simulink model "gm_ObjectTrackerHDL"  (R2024a)
settings: Solver=VariableStepAuto  StartTime=0.0  StopTime=5.5  RelTol=1e-3  EnableMultiTasking=on
PreLoadFcn:
  | % Blank input
  | img = zeros(480,640);
  | 
  | % Initialize ROI and its center
  | ROI = [175 270 127 127];
  | center = [ROI(2)+(ROI(4)+1)/2 ROI(1)+(ROI(3)+1)/2];
  | 
  | % Template Size
  | templateSize = 128;
  | tSize = templateSize;
  | 
  | % Learning rate
  | eta = 0.075;
  | 
  | % Number of training images
  | trainCount = 2;
  | 
  | % Gaussian Variance
  | sig = 2;
  | 
  | % Generate a Gaussian centered on the first frame
  | iSize = size(img);
  | [x,y] = ndgrid(1:iSize(1), 1:iSize(2));
  | gauss = exp(-((x-center(1)).^2 + (y-center(2)).^2)./(2*sig));
  | gauss = mat2gray(gauss);
  | 
  | % Generate the first template
  | img = imcrop(img, ROI);
  | gauss = imcrop(gauss, ROI);
  | 
  | % Generate the preprocess windowing function
  | [w1,w2] = meshgrid(window(@hann,tSize),window(@hann,tSize));
  | win = w1.*w2;
  | 
  | % Blank initial coefficients
  | G = zeros(tSize,tSize);
  | Ai = zeros(tSize,tSize);
  | Bi = zeros(tSize,tSize);
  | Hi = zeros(tSize,tSize);
  | 
  | numRows = tSize;
  | numCols = tSize;
InitFcn:
  | % Read the first frame
  | vidFReader = VideoReader(get_param('ObjectTrackerHDL/Input','inputFilename'));
  | img = read(vidFReader,1);
  | if (size(img,3) == 3)
  |     img = rgb2gray(img);
  | end
  | img = double(img);
  | 
  | % Initialize Object Center
  | objectCenter = str2num(get_param('ObjectTrackerHDL/ObjectTrackerHDL','objectCenter'));
  | 
  | % Template Size
  | templateSize = str2num(get_param('ObjectTrackerHDL/ObjectTrackerHDL','templateSize'));
  | originROI = objectCenter-templateSize/2;
  | tSize = templateSize;
  | 
  | % Initialize ROI and its center
  | ROI = [originROI tSize-1 tSize-1];
  | center = [ROI(2)+(ROI(4)+1)/2 ROI(1)+(ROI(3)+1)/2];
  | 
  | % Learning rate
  | eta = 0.075;
  | 
  | % Number of training images
  | trainCount = 128;
  | 
  | % Gaussian Variance
  | sig = 2;
  | 
  | % Generate a Gaussian centered on the first frame
  | iSize = size(img);
  | [x,y] = ndgrid(1:iSize(1), 1:iSize(2));
  | gauss = exp(-((x-center(1)).^2 + (y-center(2)).^2)./(2*sig));
  | gauss = mat2gray(gauss);
  | 
  | % Generate the first template
  | img = imcrop(img, ROI);
  | gauss = imcrop(gauss, ROI);
  | 
  | % Generate the preprocess windowing function
  | [w1,w2] = meshgrid(window(@hann,tSize),window(@hann,tSize));
  | win = w1.*w2;
  | 
  | % Preprocessing the first template
  | hgamma = vision.GammaCorrector(2.0,'Correction','De-gamma');
  | img = hgamma(uint8(img));
  | img = double(img);
  | mean1 = mean(img(:));
  | std1 = std(img(:));
  | img = (img-mean1)/std1;
  | fii = img.*win;
  | 
  | % Convert to frequency domain and calculate initial coefficients
  | G = fft2(gauss);
  | Ai = (G.*conj(fft2(fii)));
  | Bi = real((fft2(fii).*conj(fft2(fii))));
  | 
  | rng('default');
  | % Initial training procedure
  | for i = 1:trainCount
  |     rotateRand = 20.*rand - 10;
  |     resizeRand = 0.2.*rand + 0.9;
  |     img = imresize(imresize(imrotate(img, rotateRand), resizeRand), [tSize tSize]);
  |     img = hgamma(uint8(img));
  |     img = double(img);
  |     img = (img-mean(img(:)))/std(img(:));
  |     fii = img.*win;
  |     Ai = Ai + (G.*conj(fft2(fii)));
  |     Bi = Bi + real((fft2(fii).*conj(fft2(fii))));
  | end
  | 
  | % Initial Filter coefficients
  | Ai = eta.*Ai;
  | Bi = eta.*Bi;
  | Hi = Ai./Bi;
  | 
  | % FFT Parameters
  | numRows = tSize;
  | numCols = tSize;
model workspace (MAT data in the model file):
  mwTaskManagerKernelLatency = 0
undefined symbols (not defined in the file or in its folder): a, b, c, Rec, SDTV
libraries: hdlsllib x61, simulink x17, visionhdlutilities x8, visionstatistics x6, dsphdlxfrm2 x6, visionconversions x3, visiontransforms x3, visionhdlio x2, visionhdlconversions x2, visionhdlstatistics x2, visionsinks x1, dspvision x1
(part 1 of 3)
settings Model: SimulationMode=accelerator  Creator=The MathWorks, Inc.  LastModifiedBy=pc
settings SolverCC: PositivePriorityOrder=on
settings OptimizationCC: BlockReduction=off  ConditionallyExecuteInputs=off  DefaultParameterBehavior=Inlined  EnhancedBackFolding=on  PassReuseOutputArgsAs=Individual arguments  ZeroExternalMemoryAtStartup=off  ZeroInternalMemoryAtStartup=off  MaxStackSize=64  OptimizeBlockOrder=speed  DifferentSizesBufferReuse=on  OptimizationCustomize=off  EfficientTunableParamExpr=on
settings DebuggingCC: AlgebraicLoopMsg=error  InheritedTsInSrcMsg=none  ParameterPrecisionLossMsg=none  ParameterTunabilityLossMsg=error  FixptConstOverflowMsg=warning  SubsystemReferenceDiagnosticForUnitTest=warning
settings HardwareCC: ProdBitPerPointer=32  ProdBitPerSizeT=32  ProdBitPerPtrDiffT=32  ProdLargestAtomicFloat=None  ProdIntDivRoundTo=Undefined  ProdEndianess=Unspecified  ProdWordSize=32  ProdHWDeviceType=ASIC/FPGA->ASIC/FPGA  TargetBitPerPointer=64  TargetBitPerSizeT=64  TargetBitPerPtrDiffT=64  TargetLongLongMode=on  TargetIntDivRoundTo=Zero  TargetEndianess=LittleEndian  TargetWordSize=64  TargetHWDeviceType=Custom Processor->MATLAB Host Computer  ProdEqTarget=off  HardwareBoardFeatureSet=SoCBlockset
settings ModelReferenceCC: ModelReferenceNumInstancesAllowed=Single
settings SFSimCC: MATLABDynamicMemAlloc=off
settings RTWCC: Description=Embedded Coder  SystemTargetFile=ert.tlc  TemplateMakefile=ert_default_tmf  Toolchain=Linaro AArch64 Linux v6.3.1  GPUComputeCapability=3.5
settings CodeAppCC: ForceParamTrailComments=on  IgnoreCustomStorageClasses=off  OperatorAnnotations=on  SimulinkDataObjDesc=on  SFDataObjDesc=on  InsertBlockDesc=on
settings ERTTargetCC: ERTCustomFileTemplate=example_file_process.tlc

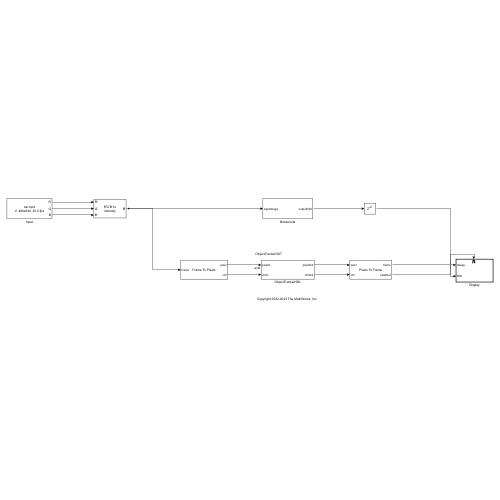
[thumbnail: Simulink's stored preview of the top-level diagram]
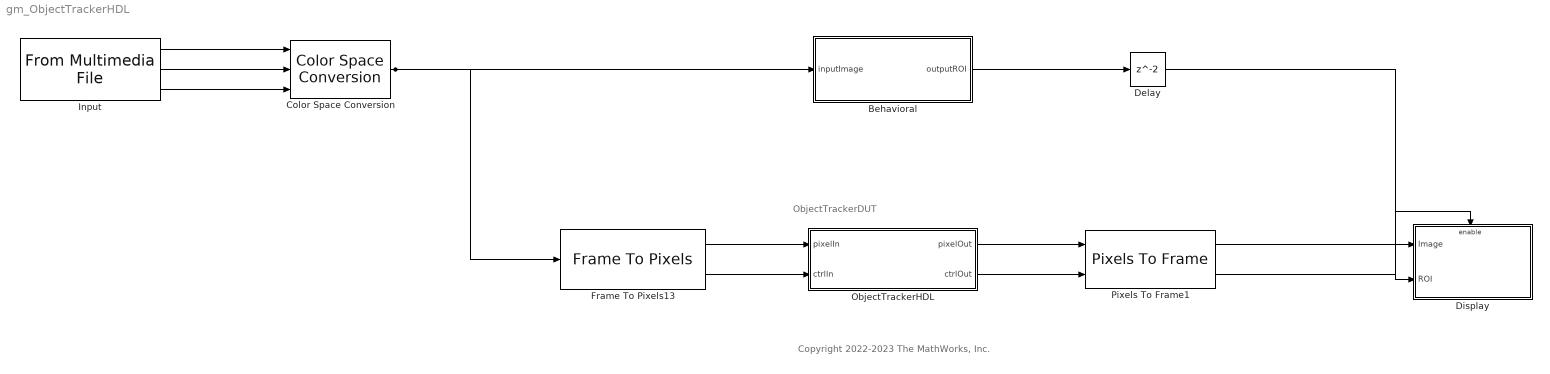
== system gm_ObjectTrackerHDL ==
  note: ObjectTrackerDUT
  note: Copyright 2022-2023 The MathWorks, Inc.
  Behavioral : Subsystem
  Color Space Conversion : visionconversions/Color Space  Conversion  conversion=Obsolete  conversionActive=R'G'B' to intensity  wp_str=D65  rec=Rec. 601 (SDTV)  sys=1125/60/2:1  imagePorts=Separate color signals
  Delay : Delay
  Display : Subsystem
  Frame To Pixels13 : visionhdlio/Frame To Pixels  NumComponents=1  NumPixels=1  VideoFormat=480p  ActivePixelsPerLine=640  ActiveVideoLines=480  TotalPixelsPerLine=800  TotalVideoLines=525  StartingActiveLine=36  FrontPorch=16  SampleTime=0  VideoFormatCache=480p  ActivePixelsPerLineCache=903  ActiveVideoLinesCache=718  TotalPixelsPerLineCache=950  TotalVideoLinesCache=750  StartingActiveLineCache=6  FrontPorchCache=5
  Input : dspvision/From Multimedia File  inputFilename=C:\Users\pc\Documents\MATLAB\Examples\R2024a\supportfiles\visionhdl\LTIR_dataset\car.mp4  readRange=[1 Inf]  loop=on  numPlays=1  outputStreams=Video only  videoDataType=uint8  audioDataType=int16  inheritSampleTime=on  userDefinedSampleTime=1  noAudioOutput=off  isIntensityVideo=off  fourcc=RGB  colorVideoFormat=Separate color signals  outputEOF=off  dataOrg=Column-major  audioFrameSize=1024  computeAudioFrameSize=off  outSamplingMode=Sample based
      settings: LibrarySourceBlock=visionsources/From Multimedia File
  ObjectTrackerHDL : Subsystem  mask{objectCenter=reshape(double([465 181]).', [1  2]), templateSize=128, imageSize=iSize}
      mask prompts: objectCenter "Object Center"; templateSize "Template Size"; imageSize "Image Size"
      mask TypeOptions templateSize: 16 | 32 | 64 | 128 | 256
  Pixels To Frame1 : visionhdlio/Pixels To Frame  NumComponents=3  NumPixels=1  VideoFormat=480p  ActivePixelsPerLine=640  ActiveVideoLines=480  TotalPixelsPerLine=800  TotalVideoLines=525  VideoFormatCache=480p  ActivePixelsPerLineCache=903  ActiveVideoLinesCache=718  TotalPixelsPerLineCache=950  TotalVideoLinesCache=750
  wires:
  Input/3 -> Color Space Conversion/3
  Input/2 -> Color Space Conversion/2
  Color Space Conversion/1 -> Frame To Pixels13/1, Behavioral/1(inputImage)
  Pixels To Frame1/1 -> Display/1(Image)
  Frame To Pixels13/2 -> ObjectTrackerHDL/2(ctrlIn)
  Input/1 -> Color Space Conversion/1
  Delay/1 -> Display/2(ROI)
  Behavioral/1(outputROI) -> Delay/1
  Pixels To Frame1/2 -> Display/Enable
  ObjectTrackerHDL/2(ctrlOut) -> Pixels To Frame1/2
  ObjectTrackerHDL/1(pixelOut) -> Pixels To Frame1/1
  Frame To Pixels13/1 -> ObjectTrackerHDL/1(pixelIn)

== system gm_ObjectTrackerHDL/Behavioral ==
  inputImage : Inport
  Preprocess : Subsystem
  Terminator : Terminator
  Track : Subsystem
  Transpose : Math  Operator=transpose
  outputROI : Outport
  wires:
  Track/2(currROI) -> Preprocess/3(currROI)
  Track/1(prevROI) -> Preprocess/2(prevROI)
  Preprocess/3(currTemplate) -> Track/2(currTemplate)
  Preprocess/2(prevTemplate) -> Track/1(prevTemplate)
  inputImage/1 -> Preprocess/1(inputImage)
  Preprocess/4(outputROI) -> Transpose/1
  Transpose/1 -> outputROI/1
  Preprocess/1(outputTemplate) -> Terminator/1

== system gm_ObjectTrackerHDL/Display ==
  Image : Inport
  ROI : Inport  Port=2
  Enable : EnablePort
  Display : visionsinks/To Video Display  windowSizeMode=True size (1:1)  openAtMdlStart=on  fullScreen=off  videoWindowX=536805376  videoWindowY=536805376  saveWindowSize=off  videoWindowWidth=1654  videoWindowHeight=1061  inputColorFormat=RGB  inputType=Obsolete  imagePorts=One multidimensional signal  OutputDevice=On-screen video monitor  dataOrg=Column-major  isWindowOpen=off
  VideoOverlay : MATLAB Function  TreatAsAtomicUnit=on
  wires:
  ROI/1 -> VideoOverlay/2(ROI)
  VideoOverlay/1(y) -> Display/1
  Image/1 -> VideoOverlay/1(img)

== system gm_ObjectTrackerHDL/ObjectTrackerHDL ==
  note: 2-D Correlation filter tracking HDL Subsystem
  pixelIn : Inport  OutDataTypeStr=uint8  PortDimensions=1  SampleTime=7.94444444444444e-08
  ctrlIn : Inport  Port=2
  Overlay : Subsystem
  Preprocess : Subsystem
  Track : Subsystem
  delayMatch : Delay  DelayLength=double(25)  InitialCondition=0  SampleTime=7.94444444444444e-08
  pixelOut : Outport  SampleTime=7.94444444444444e-08
  ctrlOut : Outport  Port=2
  wires:
  pixelIn/1 -> Overlay/1(pixelIn), Preprocess/1(pixelIn)
  ctrlIn/1 -> Overlay/2(ctrlIn), Track/5(frameCtrl), Preprocess/2(ctrlIn)
  Overlay/1(pixelOut) -> pixelOut/1
  delayMatch/1 -> ctrlOut/1
  Preprocess/5(OutputROI) -> Overlay/3(ROIIn)
  Overlay/2(ctrlOut) -> delayMatch/1
  Track/1(prevROIOut) -> Preprocess/3(prevROI)
  Track/2(currROIOut) -> Preprocess/4(currROI)
  Preprocess/1(prevPixelOut) -> Track/1(prevPixelIn)
  Preprocess/2(prevCtrlOut) -> Track/2(prevCtrlIn)
  Preprocess/3(currPixelOut) -> Track/3(currPixelIn)
  Preprocess/4(currCtrlOut) -> Track/4(currCtrlIn)

== system gm_ObjectTrackerHDL/Behavioral/Preprocess ==
  inputImage : Inport
  prevROI : Inport  Port=2
  currROI : Inport  Port=3
  Constant8 : Constant  Value=fi(win,0,16,16)  VectorParams1D=off  OutDataTypeStr=fixdt(0,16,16)  SampleTime=-1
  CurrPreprocess : Subsystem
  MATLAB Function1 : MATLAB Function  TreatAsAtomicUnit=on  mask{templateSize=tSize}
      mask prompts: templateSize "Template Size"
  MATLAB Function7 : MATLAB Function  TreatAsAtomicUnit=on  mask{templateSize=tSize}
      mask prompts: templateSize "Template Size"
  PrevPreprocess : Subsystem
  outputTemplate : Outport
  prevTemplate : Outport  Port=2
  currTemplate : Outport  Port=3
  outputROI : Outport  Port=4
  wires:
  currROI/1 -> MATLAB Function1/2(ROI)
  inputImage/1 -> MATLAB Function7/1(img), MATLAB Function1/1(img)
  prevROI/1 -> MATLAB Function7/2(ROI), outputROI/1
  PrevPreprocess/1(out) -> prevTemplate/1
  MATLAB Function1/1(fi) -> CurrPreprocess/1(in)
  Constant8/1 -> PrevPreprocess/2(window), CurrPreprocess/2(window)
  CurrPreprocess/1(out) -> currTemplate/1
  MATLAB Function7/1(fi) -> PrevPreprocess/1(in), outputTemplate/1

== system gm_ObjectTrackerHDL/Behavioral/Track ==
  prevTemplate : Inport
  currTemplate : Inport  Port=2
  2-DCorrelation : Subsystem
  MaxCorrelation : Subsystem
  ROIUpdate : Subsystem
  prevROI : Outport
  currROI : Outport  Port=2
  wires:
  2-DCorrelation/1(correlationOut) -> MaxCorrelation/1(correlationIn)
  MaxCorrelation/2(maxRow) -> ROIUpdate/2(maxRow)
  MaxCorrelation/1(maxCol) -> ROIUpdate/1(maxCol)
  prevTemplate/1 -> 2-DCorrelation/1(prevTemplate)
  ROIUpdate/1(prevROI) -> prevROI/1
  ROIUpdate/2(currROI) -> currROI/1
  currTemplate/1 -> 2-DCorrelation/2(currTemplate)

== system gm_ObjectTrackerHDL/ObjectTrackerHDL/Overlay ==
  note: Overlay Subsystem overlays the template bounding box onto the image frame
  pixelIn : Inport  OutDataTypeStr=uint8  PortDimensions=1  SampleTime=7.94444444444444e-08
  ctrlIn : Inport  Port=2
  ROIIn : Inport  Port=3  OutDataTypeStr=uint16  PortDimensions=[4]  SampleTime=7.94444444444444e-08
  Constant : Constant  OutDataTypeStr=uint16  SampleTime=7.94444444444444e-08
  ROIIn_3_term3 : Terminator
  Subtract : Sum  Inputs=+-  OutDataTypeStr=uint16  AccumDataTypeStr=uint16  SampleTime=7.94444444444444e-08
  VideoOverlay : Subsystem  mask{color=Blue, opacity=double(1), mulChannel=off, numChannel=1, planeOpacity=double(0)}
      mask prompts: opacity "Pixel Opacity"; mulChannel "Multiple Channels"; numChannel "Number of Channels"; planeOpacity "Plane Opacity"
      mask init:
      | color = double(3);
      | mulChannel = double(0);
      | numChannel = double(1);
      | opacity = double(1);
      | planeOpacity = double(0);
      mask TypeOptions color: Red | Green | Blue | Cyan | Yellow
      mask TypeOptions numChannel: 1 | 2 | 3
  concatenate : Concatenate  NumInputs=4  Mode=Multidimensional array  ConcatenateDimension=2
  t : Demux
  pixelOut : Outport  SampleTime=7.94444444444444e-08
  ctrlOut : Outport  Port=2
  wires:
  pixelIn/1 -> VideoOverlay/1(pixelIn)
  ctrlIn/1 -> VideoOverlay/2(ctrlIn)
  ROIIn/1 -> t/1
  Constant/1 -> Subtract/2
  Subtract/1 -> concatenate/4, concatenate/3
  concatenate/1 -> VideoOverlay/3(Position)
  VideoOverlay/1(pixelOut) -> pixelOut/1
  VideoOverlay/2(ctrlOut) -> ctrlOut/1
  t/1 -> concatenate/2
  t/2 -> concatenate/1
  t/3 -> Subtract/1
  t/4 -> ROIIn_3_term3/1

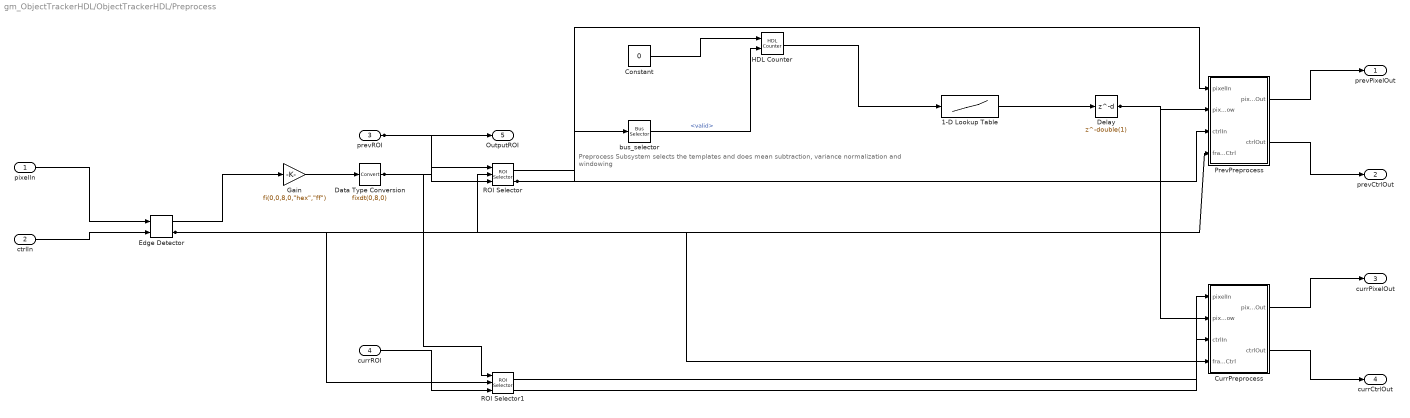
== system gm_ObjectTrackerHDL/ObjectTrackerHDL/Preprocess ==
  note: Preprocess Subsystem selects the templates and does mean subtraction, variance normalization and windowing
  pixelIn : Inport  OutDataTypeStr=uint8  PortDimensions=1  SampleTime=7.94444444444444e-08
  ctrlIn : Inport  Port=2
  prevROI : Inport  Port=3  OutDataTypeStr=uint16  PortDimensions=[4]  SampleTime=7.94444444444444e-08
  currROI : Inport  Port=4  OutDataTypeStr=uint16  PortDimensions=[4]  SampleTime=7.94444444444444e-08
  1-D Lookup Table : Lookup_n-D  NumberOfTableDimensions=1  LookupTableObject=''  BreakpointsForDimension1=[0:tSize * tSize - 1]  BreakpointsForDimension1FirstPoint=10  BreakpointsForDimension2FirstPoint=10  BreakpointsForDimension1Spacing=12  BreakpointsForDimension2Spacing=12  IndexSearchMethod=Evenly spaced points  Table=fi(win(:)',0,16,16)  InterpMethod=Flat  InternalRulePriority=Speed  OutDataTypeStr=fixdt(0,16,16)  RndMeth=Simplest
  Constant : Constant  Value=0  OutDataTypeStr=boolean  SampleTime=7.94444444444444e-08
  CurrPreprocess : Subsystem
  Data Type Conversion : DataTypeConversion  OutDataTypeStr=fixdt(0,8,0)
  Delay : Delay  DelayLength=double(1)  InitialCondition=0  SampleTime=7.94444444444444e-08
  Edge Detector : visionhdlanalysis/Edge Detector  Method=Sobel  BinaryImageOutputPort=on  GradientComponentOutputPorts=off  ThresholdSource=Property  Threshold=25  LineBufferSize=2048  PaddingMethod=Symmetric  SimulateUsing=Code generation  roundingMode=Floor  overflowMode=off  GradientMin=[]  GradientMax=[]
  Gain : Gain  Gain="fi(0,0,8,0,\"hex\",\"ff\")"  ParamDataTypeStr=fixdt(0, 8, 0)  OutDataTypeStr=uint8  SampleTime=7.94444444444444e-08
  HDL Counter : hdlsllib/Sources/HDL Counter  CountType=Count limited  CountInit=0  CountStep=1  CountMax=tSize * tSize - 1  CountFromType=Initial value  CountFrom=0  CountResetPort=on  CountLoadPort=off  CountEnbPort=on  CountDirPort=off  CountHitOutputPort=off  CountDataType=Unsigned  CountWordLen=ceil(log2(tSize * tSize - 1))  CountFracLen=0  CountSampTime=1
  PrevPreprocess : Subsystem
  ROI Selector : visionhdlutilities/ROI Selector  VerticalReuse=off  RegionsSource=Input port  NumberOfRegions=1  Regions=[100 100 50 50]  SimulateUsing=Code generation
  ROI Selector1 : visionhdlutilities/ROI Selector  VerticalReuse=off  RegionsSource=Input port  NumberOfRegions=1  Regions=[100 100 50 50]  SimulateUsing=Code generation
  bus_selector : BusSelector  OutputSignals=valid
  prevPixelOut : Outport  SampleTime=7.94444444444444e-08
  prevCtrlOut : Outport  Port=2
  currPixelOut : Outport  Port=3  SampleTime=7.94444444444444e-08
  currCtrlOut : Outport  Port=4
  OutputROI : Outport  Port=5  SampleTime=7.94444444444444e-08
  wires:
  pixelIn/1 -> Edge Detector/1
  ctrlIn/1 -> Edge Detector/2
  prevROI/1 -> OutputROI/1, ROI Selector/3
  currROI/1 -> ROI Selector1/3
  1-D Lookup Table/1 -> Delay/1
  Constant/1 -> HDL Counter/1
  CurrPreprocess/1(pixelOut) -> currPixelOut/1
  CurrPreprocess/2(ctrlOut) -> currCtrlOut/1
  Data Type Conversion/1 -> ROI Selector1/1, ROI Selector/1
  Delay/1 -> PrevPreprocess/2(pixelWindow), CurrPreprocess/2(pixelWindow)
  Edge Detector/1 -> Gain/1
  Edge Detector/2 -> PrevPreprocess/4(frameCtrl), CurrPreprocess/4(frameCtrl), ROI Selector1/2, ROI Selector/2
  Gain/1 -> Data Type Conversion/1
  HDL Counter/1 -> 1-D Lookup Table/1
  bus_selector/1 -> HDL Counter/2  "<valid>"
  PrevPreprocess/1(pixelOut) -> prevPixelOut/1
  PrevPreprocess/2(ctrlOut) -> prevCtrlOut/1
  ROI Selector/1 -> PrevPreprocess/1(pixelIn)
  ROI Selector/2 -> bus_selector/1, PrevPreprocess/3(ctrlIn)
  ROI Selector1/1 -> CurrPreprocess/1(pixelIn)
  ROI Selector1/2 -> CurrPreprocess/3(ctrlIn)

== system gm_ObjectTrackerHDL/ObjectTrackerHDL/Track ==
  note: Tracking HDL Subsystem performs 2D correlation, calculates maximum of 2D correlation point and updates the ROI
  prevPixelIn : Inport  OutDataTypeStr=fixdt(1, 32, 28)  PortDimensions=1  SampleTime=7.94444444444444e-08
  prevCtrlIn : Inport  Port=2
  currPixelIn : Inport  Port=3  OutDataTypeStr=fixdt(1, 32, 28)  PortDimensions=1  SampleTime=7.94444444444444e-08
  currCtrlIn : Inport  Port=4
  frameCtrl : Inport  Port=5
  2-DCorrelation : Subsystem
  Delay7 : Delay  DelayLength=20
  MaxCorrelation : Subsystem
  ROIUpdate : Subsystem
  prevROIOut : Outport  SampleTime=7.94444444444444e-08
  currROIOut : Outport  Port=2  SampleTime=7.94444444444444e-08
  wires:
  frameCtrl/1 -> Delay7/1, 2-DCorrelation/6(frameCtrl), MaxCorrelation/3(frameCtrl)
  ROIUpdate/2(prevROI) -> prevROIOut/1
  ROIUpdate/3(currROI) -> currROIOut/1
  2-DCorrelation/1(pixelOut) -> MaxCorrelation/1(pixelIn)
  MaxCorrelation/1(maxCol) -> ROIUpdate/1(maxCol)
  2-DCorrelation/2(ctrlOut) -> MaxCorrelation/2(ctrlIn)
  prevPixelIn/1 -> 2-DCorrelation/1(prevPixelIn)
  prevCtrlIn/1 -> 2-DCorrelation/2(prevCtrlIn)
  currPixelIn/1 -> 2-DCorrelation/3(currPixelIn)
  currCtrlIn/1 -> 2-DCorrelation/4(currCtrlIn)
  MaxCorrelation/2(maxRow) -> ROIUpdate/2(maxRow)
  ROIUpdate/1(streamCtrlOut) -> 2-DCorrelation/5(streamCtrlIn)
  Delay7/1 -> ROIUpdate/3(frameCtrl)

== system gm_ObjectTrackerHDL/Behavioral/Preprocess/CurrPreprocess ==
  in : Inport
  window : Inport  Port=2
  2-D Mean2 : visionstatistics/2-D Mean  run=off  reset_popup=None  directionMode=Entire input  dimension=1  treatSBRowAsCol=on  outputMode=Binary point scaling  outputWordLength=8  outputFracLength=0  outputLastDataTypeStr=fixdt([],8,0)  accumMode=Binary point scaling  accumWordLength=32  accumFracLength=0  accumLastDataTypeStr=fixdt([],32,0)  roiEnable=off  roiType=Rectangles  roiPortion=Entire ROI  roiOutput=Individual statistics for each ROI  roiFlag=off  roundingMode=Floor  overflowMode=on  accumDataTypeStr=fixdt([],32,0)  outputDataTypeStr=fixdt([],8,0)  outputMin=[]  outputMax=[]
  2-D Standard Deviation : visionstatistics/2-D Standard Deviation  run=off  reset_popup=None  InputProcessing=Columns as channels (frame based)  directionMode=Entire input  dimension=1  treatSBRowAsCol=on  roiEnable=off  roiType=Rectangles  roiPortion=Entire ROI  roiOutput=Individual statistics for each ROI  roiFlag=off
  Data Type Conversion2 : DataTypeConversion  OutDataTypeStr=uint8  SaturateOnIntegerOverflow=off  RndMeth=Floor
  Data Type Conversion3 : DataTypeConversion  OutDataTypeStr=single  SaturateOnIntegerOverflow=off  RndMeth=Floor
  Delay : Delay  DelayLength=1  InitialCondition=uint8(mean1)
  Delay1 : Delay  DelayLength=1  InitialCondition=uint8(std1)
  Divide1 : Product  Inputs=*/  OutDataTypeStr=fixdt(1,16,12)  SaturateOnIntegerOverflow=on
  Gamma Correction : visionconversions/Gamma Correction  operation=De-gamma  gamma=2  linearSegment=on  breakPoint=0.018
  Product : Product
  Subtract2 : Sum  Inputs=+-  OutDataTypeStr=fixdt(1,16,0)
  out : Outport
  wires:
  Delay/1 -> Subtract2/2
  Delay1/1 -> Divide1/2
  Product/1 -> out/1
  window/1 -> Product/2
  Subtract2/1 -> Divide1/1
  Data Type Conversion3/1 -> 2-D Standard Deviation/1
  2-D Mean2/1 -> Delay/1
  Divide1/1 -> Product/1
  in/1 -> Gamma Correction/1
  Data Type Conversion2/1 -> Delay1/1
  2-D Standard Deviation/1 -> Data Type Conversion2/1
  Gamma Correction/1 -> Subtract2/1, 2-D Mean2/1, Data Type Conversion3/1

== system gm_ObjectTrackerHDL/Behavioral/Preprocess/PrevPreprocess ==
  in : Inport
  window : Inport  Port=2
  2-D Mean2 : visionstatistics/2-D Mean  run=off  reset_popup=None  directionMode=Entire input  dimension=1  treatSBRowAsCol=on  outputMode=Binary point scaling  outputWordLength=8  outputFracLength=0  outputLastDataTypeStr=fixdt([],8,0)  accumMode=Binary point scaling  accumWordLength=32  accumFracLength=0  accumLastDataTypeStr=fixdt([],32,0)  roiEnable=off  roiType=Rectangles  roiPortion=Entire ROI  roiOutput=Individual statistics for each ROI  roiFlag=off  roundingMode=Floor  overflowMode=on  accumDataTypeStr=fixdt([],32,0)  outputDataTypeStr=fixdt([],8,0)  outputMin=[]  outputMax=[]
  2-D Standard Deviation : visionstatistics/2-D Standard Deviation  run=off  reset_popup=None  InputProcessing=Columns as channels (frame based)  directionMode=Entire input  dimension=1  treatSBRowAsCol=on  roiEnable=off  roiType=Rectangles  roiPortion=Entire ROI  roiOutput=Individual statistics for each ROI  roiFlag=off
  Data Type Conversion2 : DataTypeConversion  OutDataTypeStr=uint8  SaturateOnIntegerOverflow=off  RndMeth=Floor
  Data Type Conversion3 : DataTypeConversion  OutDataTypeStr=single  SaturateOnIntegerOverflow=off  RndMeth=Floor
  Delay : Delay  DelayLength=1  InitialCondition=uint8(mean1)
  Delay1 : Delay  DelayLength=1  InitialCondition=uint8(std1)
  Divide1 : Product  Inputs=*/  OutDataTypeStr=fixdt(1,16,12)  SaturateOnIntegerOverflow=on
  Gamma Correction : visionconversions/Gamma Correction  operation=De-gamma  gamma=2  linearSegment=on  breakPoint=0.018
  Product : Product
  Subtract2 : Sum  Inputs=+-  OutDataTypeStr=fixdt(1,16,0)
  out : Outport
  wires:
  Delay1/1 -> Divide1/2
  Delay/1 -> Subtract2/2
  Product/1 -> out/1
  window/1 -> Product/2
  Subtract2/1 -> Divide1/1
  Data Type Conversion3/1 -> 2-D Standard Deviation/1
  2-D Mean2/1 -> Delay/1
  Divide1/1 -> Product/1
  in/1 -> Gamma Correction/1
  Data Type Conversion2/1 -> Delay1/1
  2-D Standard Deviation/1 -> Data Type Conversion2/1
  Gamma Correction/1 -> Subtract2/1, 2-D Mean2/1, Data Type Conversion3/1

== system gm_ObjectTrackerHDL/Behavioral/Track/2-DCorrelation ==
  prevTemplate : Inport
  currTemplate : Inport  Port=2
  2-D FFT : visiontransforms/2-D FFT  TableOpt=NEW  TableOptActive=Speed  FFTImplementation=Auto  BitRevOrder=off  SkipNorm=off  firstCoeffLastDataTypeStr=Inherit: Same word length as input  outputMode=Binary point scaling  outputWordLength=24  outputFracLength=12  outputLastDataTypeStr=fixdt(1,24,12)  roundingMode=Floor  overflowMode=off  firstCoeffDataTypeStr=Inherit: Same word length as input  outputDataTypeStr=fixdt(1,24,12)  outputMin=[]  outputMax=[]
  2-D FFT1 : visiontransforms/2-D FFT  TableOpt=NEW  TableOptActive=Speed  FFTImplementation=Auto  BitRevOrder=off  SkipNorm=off  firstCoeffLastDataTypeStr=Inherit: Same word length as input  outputMode=Binary point scaling  outputWordLength=24  outputFracLength=12  outputLastDataTypeStr=fixdt(1,24,12)  roundingMode=Floor  overflowMode=off  firstCoeffDataTypeStr=Inherit: Same word length as input  outputDataTypeStr=fixdt(1,24,12)  outputMin=[]  outputMax=[]
  2-D IFFT : visiontransforms/2-D IFFT  TableOpt=NEW  TableOptActive=Speed  FFTImplementation=Auto  BitRevOrder=off  cs_in=off  divideOutput=on  SkipNorm=on  firstCoeffLastDataTypeStr=Inherit: Same word length as input  outputMode=Binary point scaling  outputWordLength=24  outputFracLength=16  outputLastDataTypeStr=fixdt(1,24,16)  roundingMode=Floor  overflowMode=off  firstCoeffDataTypeStr=Inherit: Same word length as input  outputDataTypeStr=fixdt(1,24,16)  outputMin=[]  outputMax=[]
  CoefficientsUpdate : Subsystem
  Product8 : Product  OutDataTypeStr=fixdt(1,24,16)
  Transpose : Math  Operator=transpose
  Transpose1 : Math  Operator=transpose
  Transpose2 : Math  Operator=transpose
  correlationOut : Outport
  wires:
  Transpose2/1 -> correlationOut/1
  Transpose1/1 -> CoefficientsUpdate/1(In)
  2-D FFT1/1 -> Transpose1/1
  currTemplate/1 -> 2-D FFT1/1
  Transpose/1 -> Product8/1
  2-D IFFT/1 -> Transpose2/1
  Product8/1 -> 2-D IFFT/1
  2-D FFT/1 -> Transpose/1
  CoefficientsUpdate/1(Out) -> Product8/2
  prevTemplate/1 -> 2-D FFT/1

== system gm_ObjectTrackerHDL/Behavioral/Track/MaxCorrelation ==
  correlationIn : Inport
  2-D Mean3 : visionstatistics/2-D Mean  run=off  reset_popup=None  directionMode=Entire input  dimension=1  treatSBRowAsCol=on  outputLastDataTypeStr=Inherit: Same as accumulator  accumMode=Binary point scaling  accumWordLength=16  accumFracLength=0  accumLastDataTypeStr=fixdt([],16,0)  roiEnable=off  roiType=Rectangles  roiPortion=Entire ROI  roiOutput=Individual statistics for each ROI  roiFlag=off  roundingMode=Floor  overflowMode=off  accumDataTypeStr=fixdt([],16,0)  outputDataTypeStr=Inherit: Same as accumulator  outputMin=[]  outputMax=[]
  2-D Mean4 : visionstatistics/2-D Mean  run=off  reset_popup=None  directionMode=Entire input  dimension=1  treatSBRowAsCol=on  outputLastDataTypeStr=Inherit: Same as accumulator  accumMode=Binary point scaling  accumWordLength=16  accumFracLength=0  accumLastDataTypeStr=fixdt([],16,0)  roiEnable=off  roiType=Rectangles  roiPortion=Entire ROI  roiOutput=Individual statistics for each ROI  roiFlag=off  roundingMode=Floor  overflowMode=off  accumDataTypeStr=fixdt([],16,0)  outputDataTypeStr=Inherit: Same as accumulator  outputMin=[]  outputMax=[]
  Complex to Real-Imag : ComplexToRealImag
  Data Type Conversion1 : DataTypeConversion  OutDataTypeStr=uint16  SaturateOnIntegerOverflow=off  RndMeth=Floor
  Data Type Conversion3 : DataTypeConversion  OutDataTypeStr=single  SaturateOnIntegerOverflow=off  RndMeth=Floor
  Data Type Conversion4 : DataTypeConversion  OutDataTypeStr=uint16  SaturateOnIntegerOverflow=off  RndMeth=Floor
  MATLAB Function13 : MATLAB Function  TreatAsAtomicUnit=on
  Terminator : Terminator
  maxCol : Outport
  maxRow : Outport  Port=2
  wires:
  correlationIn/1 -> Data Type Conversion3/1
  2-D Mean4/1 -> maxRow/1
  MATLAB Function13/1(P) -> Data Type Conversion1/1
  2-D Mean3/1 -> maxCol/1
  Data Type Conversion3/1 -> Complex to Real-Imag/1
  Data Type Conversion1/1 -> 2-D Mean3/1
  Data Type Conversion4/1 -> 2-D Mean4/1
  MATLAB Function13/2(Q) -> Data Type Conversion4/1
  Complex to Real-Imag/2 -> Terminator/1
  Complex to Real-Imag/1 -> MATLAB Function13/1(gi)

== system gm_ObjectTrackerHDL/Behavioral/Track/ROIUpdate ==
  maxCol : Inport
  maxRow : Inport  Port=2
  Add4 : Sum  OutDataTypeStr=uint16
  Add5 : Sum  OutDataTypeStr=uint16
  CurrValidROI : Subsystem
  Delay7 : Delay  DelayLength=1  InitialConditionSource=Input port  InitialCondition=0
      settings: InputPortMap=u0,p4
  Demux1 : Demux
  Mux1 : Mux
  PrevValidROI : Subsystem
  ROI : Constant  Value=uint16(ROI)  OutDataTypeStr=uint16  SampleTime=-1
  Subtract3 : Sum  Inputs=+-  OutDataTypeStr=fixdt(1,17,0)
  Subtract4 : Sum  Inputs=+-  OutDataTypeStr=fixdt(1,17,0)
  height/2 : Constant  Value=uint16(tSize/2)  SampleTime=-1
  width/2 : Constant  Value=uint16(tSize/2)  SampleTime=-1
  prevROI : Outport
  currROI : Outport  Port=2
  wires:
  Mux1/1 -> CurrValidROI/1(ROIIn), Delay7/1
  Delay7/1 -> Demux1/1, PrevValidROI/1(ROIIn)
  ROI/1 -> Delay7/2
  CurrValidROI/1(ROIOut) -> currROI/1
  PrevValidROI/1(ROIOut) -> prevROI/1
  maxRow/1 -> Subtract4/1
  Demux1/1 -> Add5/2
  Subtract3/1 -> Add4/1
  Add5/1 -> Mux1/1
  Add4/1 -> Mux1/2
  width/2/1 -> Subtract4/2
  Subtract4/1 -> Add5/1
  Demux1/4 -> Mux1/4
  Demux1/3 -> Mux1/3
  Demux1/2 -> Add4/2
  height/2/1 -> Subtract3/2
  maxCol/1 -> Subtract3/1

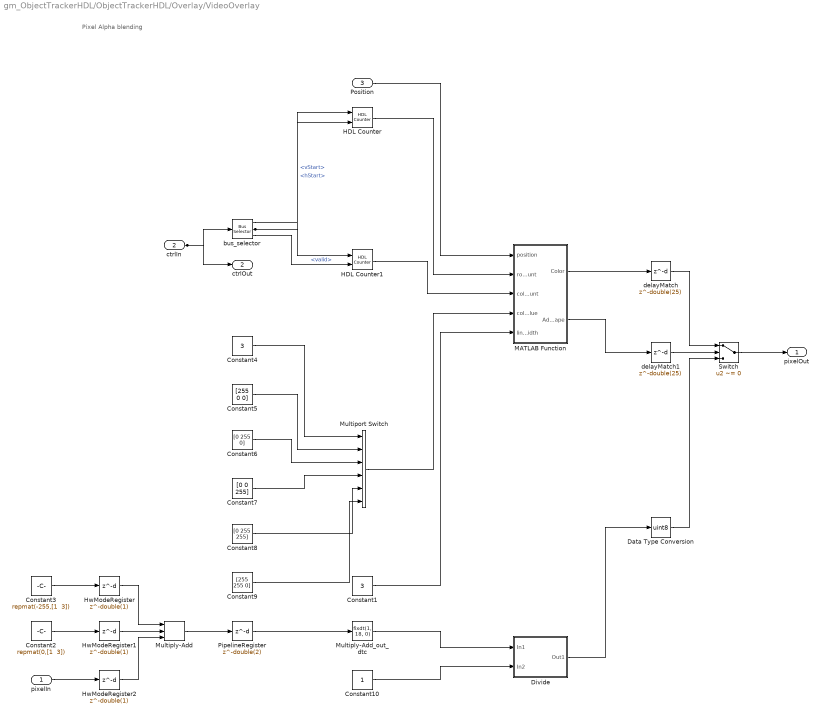
== system gm_ObjectTrackerHDL/ObjectTrackerHDL/Overlay/VideoOverlay ==
  note: Pixel Alpha blending
  pixelIn : Inport  OutDataTypeStr=uint8  PortDimensions=1  SampleTime=7.94444444444444e-08
  ctrlIn : Inport  Port=2
  Position : Inport  Port=3  OutDataTypeStr=uint16  PortDimensions=[1 4]  SampleTime=7.94444444444444e-08
  Constant1 : Constant  Value=3  VectorParams1D=off  OutDataTypeStr=uint8  SampleTime=7.94444444444444e-08
  Constant10 : Constant  VectorParams1D=off  OutDataTypeStr=int8  SampleTime=7.94444444444444e-08
  Constant2 : Constant  Value="repmat(0,[1  3])"  VectorParams1D=off  OutDataTypeStr=int8  SampleTime=7.94444444444444e-08
  Constant3 : Constant  Value="repmat(-255,[1  3])"  VectorParams1D=off  OutDataTypeStr=fixdt(1, 9, 0)  SampleTime=7.94444444444444e-08
  Constant4 : Constant  Value=3  OutDataTypeStr=uint8  SampleTime=7.94444444444444e-08
  Constant5 : Constant  Value=[255 0 0]  VectorParams1D=off  OutDataTypeStr=uint8  SampleTime=7.94444444444444e-08
  Constant6 : Constant  Value=[0 255 0]  VectorParams1D=off  OutDataTypeStr=uint8  SampleTime=7.94444444444444e-08
  Constant7 : Constant  Value=[0 0 255]  VectorParams1D=off  OutDataTypeStr=uint8  SampleTime=7.94444444444444e-08
  Constant8 : Constant  Value=[0 255 255]  VectorParams1D=off  OutDataTypeStr=uint8  SampleTime=7.94444444444444e-08
  Constant9 : Constant  Value=[255 255 0]  VectorParams1D=off  OutDataTypeStr=uint8  SampleTime=7.94444444444444e-08
  Data Type Conversion : DataTypeConversion  OutDataTypeStr=uint8  SampleTime=7.94444444444444e-08  SaturateOnIntegerOverflow=off  RndMeth=Floor
  Divide : Subsystem
  HDL Counter : hdlsllib/Sources/HDL Counter  CountType=Free running  CountInit=0  CountStep=1  CountMax=240  CountFromType=Initial value  CountFrom=0  CountResetPort=on  CountLoadPort=off  CountEnbPort=on  CountDirPort=off  CountHitOutputPort=off  CountDataType=Signed  CountWordLen=32  CountFracLen=0  CountSampTime=1
  HDL Counter1 : hdlsllib/Sources/HDL Counter  CountType=Free running  CountInit=0  CountStep=1  CountMax=360  CountFromType=Initial value  CountFrom=0  CountResetPort=on  CountLoadPort=off  CountEnbPort=on  CountDirPort=off  CountHitOutputPort=off  CountDataType=Signed  CountWordLen=32  CountFracLen=0  CountSampTime=1
  HwModeRegister : Delay  DelayLength=double(1)  InitialCondition=0  SampleTime=7.94444444444444e-08
  HwModeRegister1 : Delay  DelayLength=double(1)  InitialCondition=0  SampleTime=7.94444444444444e-08
  HwModeRegister2 : Delay  DelayLength=double(1)  InitialCondition=0  SampleTime=7.94444444444444e-08
  MATLAB Function : Subsystem
  Multiply-Add : hdlsllib/HDL Operations/Multiply-Add  Function=c+(a.*b)  datatype=fixdt(1, 19, 0)  DoSatur=off  FMA=off
  Multiply-Add_out_dtc : DataTypeConversion  OutDataTypeStr=fixdt(1, 18, 0)  SampleTime=7.94444444444444e-08  SaturateOnIntegerOverflow=off  RndMeth=Floor
  Multiport Switch : MultiPortSwitch  Inputs=5  DiagnosticForDefault=None  OutDataTypeStr=uint8  SampleTime=7.94444444444444e-08  SaturateOnIntegerOverflow=off  InputSameDT=off
  PipelineRegister : Delay  DelayLength=double(2)  InitialCondition=0  SampleTime=7.94444444444444e-08
  Switch : Switch  Criteria=u2 ~= 0  Threshold=double(0)  OutDataTypeStr=uint8  SampleTime=7.94444444444444e-08  SaturateOnIntegerOverflow=off  InputSameDT=off
  bus_selector : BusSelector  OutputSignals=vStart,hStart,valid
  delayMatch : Delay  DelayLength=double(25)  InitialCondition=0  SampleTime=7.94444444444444e-08
  delayMatch1 : Delay  DelayLength=double(25)  InitialCondition=0  SampleTime=7.94444444444444e-08
  pixelOut : Outport  SampleTime=7.94444444444444e-08
  ctrlOut : Outport  Port=2
  wires:
  pixelIn/1 -> HwModeRegister2/1
  ctrlIn/1 -> bus_selector/1, ctrlOut/1
  Position/1 -> MATLAB Function/1(position)
  bus_selector/1 -> HDL Counter/1  "<vStart>"
  bus_selector/2 -> HDL Counter1/1, HDL Counter/2  "<hStart>"
  bus_selector/3 -> HDL Counter1/2  "<valid>"
  Constant1/1 -> MATLAB Function/5(lineWidth)
  Constant10/1 -> Divide/2(In2)
  Constant2/1 -> HwModeRegister1/1
  Constant3/1 -> HwModeRegister/1
  Constant4/1 -> Multiport Switch/1
  Constant5/1 -> Multiport Switch/2
  Constant6/1 -> Multiport Switch/3
  Constant7/1 -> Multiport Switch/4
  Constant8/1 -> Multiport Switch/5
  Constant9/1 -> Multiport Switch/6
  Data Type Conversion/1 -> Switch/3
  Divide/1(Out1) -> Data Type Conversion/1
  HDL Counter/1 -> MATLAB Function/2(rowCount)
  HDL Counter1/1 -> MATLAB Function/3(colCount)
  delayMatch/1 -> Switch/1
  delayMatch1/1 -> Switch/2
  Multiply-Add_out_dtc/1 -> Divide/1(In1)
  Multiport Switch/1 -> MATLAB Function/4(colorValue)
  Switch/1 -> pixelOut/1
  PipelineRegister/1 -> Multiply-Add_out_dtc/1
  MATLAB Function/1(Color) -> delayMatch/1
  MATLAB Function/2(AddShape) -> delayMatch1/1
  Multiply-Add/1 -> PipelineRegister/1
  HwModeRegister/1 -> Multiply-Add/1
  HwModeRegister1/1 -> Multiply-Add/2
  HwModeRegister2/1 -> Multiply-Add/3

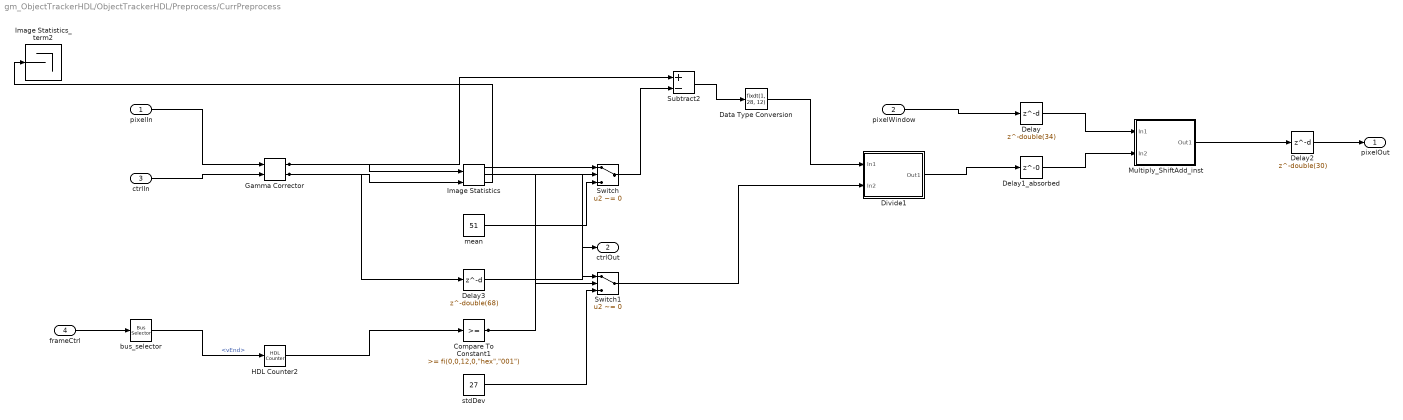
== system gm_ObjectTrackerHDL/ObjectTrackerHDL/Preprocess/CurrPreprocess ==
  pixelIn : Inport  OutDataTypeStr=uint8  PortDimensions=1  SampleTime=7.94444444444444e-08
  pixelWindow : Inport  Port=2  OutDataTypeStr=fixdt(0, 16, 16)  PortDimensions=1  SampleTime=7.94444444444444e-08
  ctrlIn : Inport  Port=3
  frameCtrl : Inport  Port=4
  Compare To Constant1 : simulink/Logic and Bit Operations/Compare To Constant  relop=>=  const="fi(0,0,12,0,\"hex\",\"001\")"  OutDataTypeStr=boolean
  Data Type Conversion : DataTypeConversion  OutDataTypeStr=fixdt(1, 28, 12)  SampleTime=7.94444444444444e-08  SaturateOnIntegerOverflow=off  RndMeth=Floor
  Delay : Delay  DelayLength=double(34)  InitialCondition=0  SampleTime=7.94444444444444e-08
  Delay1_absorbed : Delay  DelayLength=0
  Delay2 : Delay  DelayLength=double(30)  InitialCondition=0  SampleTime=7.94444444444444e-08
  Delay3 : Delay  DelayLength=double(68)  SampleTime=7.94444444444444e-08
  Divide1 : Subsystem
  Gamma Corrector : visionhdlconversions/Gamma Corrector  Correction=De-gamma  Gamma=2  LinearSegment=on  BreakPoint=0.018  SimulateUsing=Code generation
  HDL Counter2 : hdlsllib/Sources/HDL Counter  CountType=Count limited  CountInit=0  CountStep=1  CountMax=4095  CountFromType=Initial value  CountFrom=0  CountResetPort=off  CountLoadPort=off  CountEnbPort=on  CountDirPort=off  CountHitOutputPort=off  CountDataType=Unsigned  CountWordLen=12  CountFracLen=0  CountSampTime=1
  Image Statistics : visionhdlstatistics/Image Statistics  mean=on  variance=off  stdDev=on  SimulateUsing=Code generation
  Image Statistics_term2 : Terminator
  Multiply_ShiftAdd_inst : Subsystem
  Subtract2 : Sum  Inputs=+-  OutDataTypeStr=int16  AccumDataTypeStr=fixdt(1, 9, 0)  SampleTime=7.94444444444444e-08
  Switch : Switch  Criteria=u2 ~= 0  Threshold=double(0)  OutDataTypeStr=uint8  SampleTime=7.94444444444444e-08  SaturateOnIntegerOverflow=off  InputSameDT=off
  Switch1 : Switch  Criteria=u2 ~= 0  Threshold=double(0)  OutDataTypeStr=uint8  SampleTime=7.94444444444444e-08  SaturateOnIntegerOverflow=off  InputSameDT=off
  bus_selector : BusSelector  OutputSignals=vEnd
  mean : Constant  Value=51  OutDataTypeStr=uint8  SampleTime=7.94444444444444e-08
  stdDev : Constant  Value=27  OutDataTypeStr=uint8  SampleTime=7.94444444444444e-08
  pixelOut : Outport  SampleTime=7.94444444444444e-08
  ctrlOut : Outport  Port=2
  wires:
  pixelIn/1 -> Gamma Corrector/1
  pixelWindow/1 -> Delay/1
  ctrlIn/1 -> Gamma Corrector/2
  frameCtrl/1 -> bus_selector/1
  Compare To Constant1/1 -> Switch1/2, Switch/2
  Data Type Conversion/1 -> Divide1/1(In1)
  Delay/1 -> Multiply_ShiftAdd_inst/1(In1)
  Delay1_absorbed/1 -> Multiply_ShiftAdd_inst/2(In2)
  Delay2/1 -> pixelOut/1
  Delay3/1 -> ctrlOut/1
  Gamma Corrector/1 -> Subtract2/1, Image Statistics/1
  Gamma Corrector/2 -> Delay3/1, Image Statistics/2
  HDL Counter2/1 -> Compare To Constant1/1
  Image Statistics/1 -> Switch/1
  Image Statistics/2 -> Switch1/1
  Image Statistics/3 -> Image Statistics_term2/1
  bus_selector/1 -> HDL Counter2/1  "<vEnd>"
  Multiply_ShiftAdd_inst/1(Out1) -> Delay2/1
  Subtract2/1 -> Data Type Conversion/1
  Switch/1 -> Subtract2/2
  Switch1/1 -> Divide1/2(In2)
  mean/1 -> Switch/3
  stdDev/1 -> Switch1/3
  Divide1/1(Out1) -> Delay1_absorbed/1

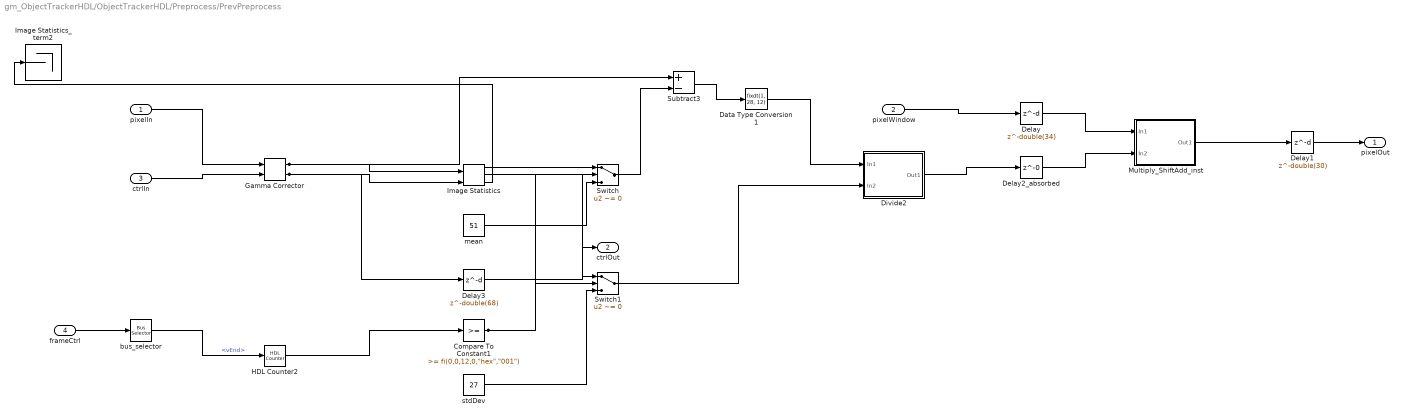
== system gm_ObjectTrackerHDL/ObjectTrackerHDL/Preprocess/PrevPreprocess ==
  pixelIn : Inport  OutDataTypeStr=uint8  PortDimensions=1  SampleTime=7.94444444444444e-08
  pixelWindow : Inport  Port=2  OutDataTypeStr=fixdt(0, 16, 16)  PortDimensions=1  SampleTime=7.94444444444444e-08
  ctrlIn : Inport  Port=3
  frameCtrl : Inport  Port=4
  Compare To Constant1 : simulink/Logic and Bit Operations/Compare To Constant  relop=>=  const="fi(0,0,12,0,\"hex\",\"001\")"  OutDataTypeStr=boolean
  Data Type Conversion1 : DataTypeConversion  OutDataTypeStr=fixdt(1, 28, 12)  SampleTime=7.94444444444444e-08  SaturateOnIntegerOverflow=off  RndMeth=Floor
  Delay : Delay  DelayLength=double(34)  InitialCondition=0  SampleTime=7.94444444444444e-08
  Delay1 : Delay  DelayLength=double(30)  InitialCondition=0  SampleTime=7.94444444444444e-08
  Delay2_absorbed : Delay  DelayLength=0
  Delay3 : Delay  DelayLength=double(68)  SampleTime=7.94444444444444e-08
  Divide2 : Subsystem
  Gamma Corrector : visionhdlconversions/Gamma Corrector  Correction=De-gamma  Gamma=2  LinearSegment=on  BreakPoint=0.018  SimulateUsing=Code generation
  HDL Counter2 : hdlsllib/Sources/HDL Counter  CountType=Count limited  CountInit=0  CountStep=1  CountMax=4095  CountFromType=Initial value  CountFrom=0  CountResetPort=off  CountLoadPort=off  CountEnbPort=on  CountDirPort=off  CountHitOutputPort=off  CountDataType=Unsigned  CountWordLen=12  CountFracLen=0  CountSampTime=1
  Image Statistics : visionhdlstatistics/Image Statistics  mean=on  variance=off  stdDev=on  SimulateUsing=Code generation
  Image Statistics_term2 : Terminator
  Multiply_ShiftAdd_inst : Subsystem
  Subtract3 : Sum  Inputs=+-  OutDataTypeStr=int16  AccumDataTypeStr=fixdt(1, 9, 0)  SampleTime=7.94444444444444e-08
  Switch : Switch  Criteria=u2 ~= 0  Threshold=double(0)  OutDataTypeStr=uint8  SampleTime=7.94444444444444e-08  SaturateOnIntegerOverflow=off  InputSameDT=off
  Switch1 : Switch  Criteria=u2 ~= 0  Threshold=double(0)  OutDataTypeStr=uint8  SampleTime=7.94444444444444e-08  SaturateOnIntegerOverflow=off  InputSameDT=off
  bus_selector : BusSelector  OutputSignals=vEnd
  mean : Constant  Value=51  OutDataTypeStr=uint8  SampleTime=7.94444444444444e-08
  stdDev : Constant  Value=27  OutDataTypeStr=uint8  SampleTime=7.94444444444444e-08
  pixelOut : Outport  SampleTime=7.94444444444444e-08
  ctrlOut : Outport  Port=2
  wires:
  pixelIn/1 -> Gamma Corrector/1
  pixelWindow/1 -> Delay/1
  ctrlIn/1 -> Gamma Corrector/2
  frameCtrl/1 -> bus_selector/1
  Compare To Constant1/1 -> Switch1/2, Switch/2
  Data Type Conversion1/1 -> Divide2/1(In1)
  Delay/1 -> Multiply_ShiftAdd_inst/1(In1)
  Delay1/1 -> pixelOut/1
  Delay2_absorbed/1 -> Multiply_ShiftAdd_inst/2(In2)
  Delay3/1 -> ctrlOut/1
  Gamma Corrector/1 -> Subtract3/1, Image Statistics/1
  Gamma Corrector/2 -> Delay3/1, Image Statistics/2
  HDL Counter2/1 -> Compare To Constant1/1
  Image Statistics/1 -> Switch/1
  Image Statistics/2 -> Switch1/1
  Image Statistics/3 -> Image Statistics_term2/1
  bus_selector/1 -> HDL Counter2/1  "<vEnd>"
  Multiply_ShiftAdd_inst/1(Out1) -> Delay1/1
  Subtract3/1 -> Data Type Conversion1/1
  Switch/1 -> Subtract3/2
  Switch1/1 -> Divide2/2(In2)
  mean/1 -> Switch/3
  stdDev/1 -> Switch1/3
  Divide2/1(Out1) -> Delay2_absorbed/1

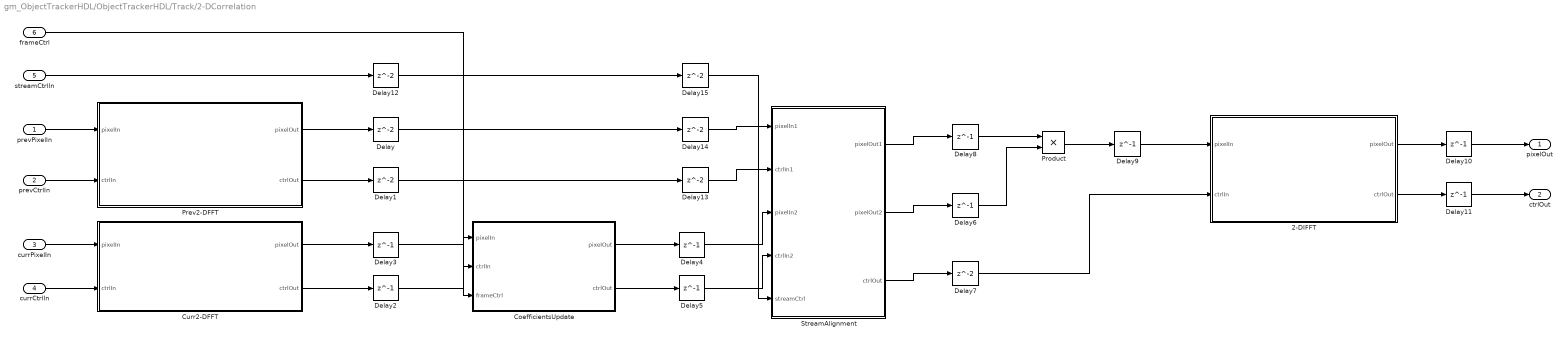
== system gm_ObjectTrackerHDL/ObjectTrackerHDL/Track/2-DCorrelation ==
  prevPixelIn : Inport  OutDataTypeStr=fixdt(1, 32, 28)  PortDimensions=1  SampleTime=7.94444444444444e-08
  prevCtrlIn : Inport  Port=2
  currPixelIn : Inport  Port=3  OutDataTypeStr=fixdt(1, 32, 28)  PortDimensions=1  SampleTime=7.94444444444444e-08
  currCtrlIn : Inport  Port=4
  streamCtrlIn : Inport  Port=5  OutDataTypeStr=boolean  PortDimensions=1  SampleTime=7.94444444444444e-08
  frameCtrl : Inport  Port=6
  2-DIFFT : Subsystem
  CoefficientsUpdate : Subsystem
  Curr2-DFFT : Subsystem
  Delay{,1,7,12..15} (7 alike) : Delay
  Delay{2..6,8..11} (9 alike) : Delay  DelayLength=1
  Prev2-DFFT : Subsystem
  Product : Product  OutDataTypeStr=fixdt(1,24,16)
  StreamAlignment : Subsystem
  pixelOut : Outport  SampleTime=7.94444444444444e-08
  ctrlOut : Outport  Port=2
  wires:
  prevPixelIn/1 -> Prev2-DFFT/1(pixelIn)
  prevCtrlIn/1 -> Prev2-DFFT/2(ctrlIn)
  currPixelIn/1 -> Curr2-DFFT/1(pixelIn)
  currCtrlIn/1 -> Curr2-DFFT/2(ctrlIn)
  streamCtrlIn/1 -> Delay12/1
  frameCtrl/1 -> CoefficientsUpdate/3(frameCtrl)
  2-DIFFT/1(pixelOut) -> Delay10/1
  2-DIFFT/2(ctrlOut) -> Delay11/1
  CoefficientsUpdate/1(pixelOut) -> Delay4/1
  CoefficientsUpdate/2(ctrlOut) -> Delay5/1
  Curr2-DFFT/1(pixelOut) -> Delay3/1
  Curr2-DFFT/2(ctrlOut) -> Delay2/1
  Delay/1 -> Delay14/1
  Delay1/1 -> Delay13/1
  Delay10/1 -> pixelOut/1
  Delay11/1 -> ctrlOut/1
  Delay12/1 -> Delay15/1
  Delay13/1 -> StreamAlignment/2(ctrlIn1)
  Delay14/1 -> StreamAlignment/1(pixelIn1)
  Delay15/1 -> StreamAlignment/5(streamCtrl)
  Delay2/1 -> CoefficientsUpdate/2(ctrlIn)
  Delay3/1 -> CoefficientsUpdate/1(pixelIn)
  Delay4/1 -> StreamAlignment/3(pixelIn2)
  Delay5/1 -> StreamAlignment/4(ctrlIn2)
  Delay6/1 -> Product/2
  Delay7/1 -> 2-DIFFT/2(ctrlIn)
  Delay8/1 -> Product/1
  Delay9/1 -> 2-DIFFT/1(pixelIn)
  Prev2-DFFT/1(pixelOut) -> Delay/1
  Prev2-DFFT/2(ctrlOut) -> Delay1/1
  Product/1 -> Delay9/1
  StreamAlignment/1(pixelOut1) -> Delay8/1
  StreamAlignment/2(pixelOut2) -> Delay6/1
  StreamAlignment/3(ctrlOut) -> Delay7/1

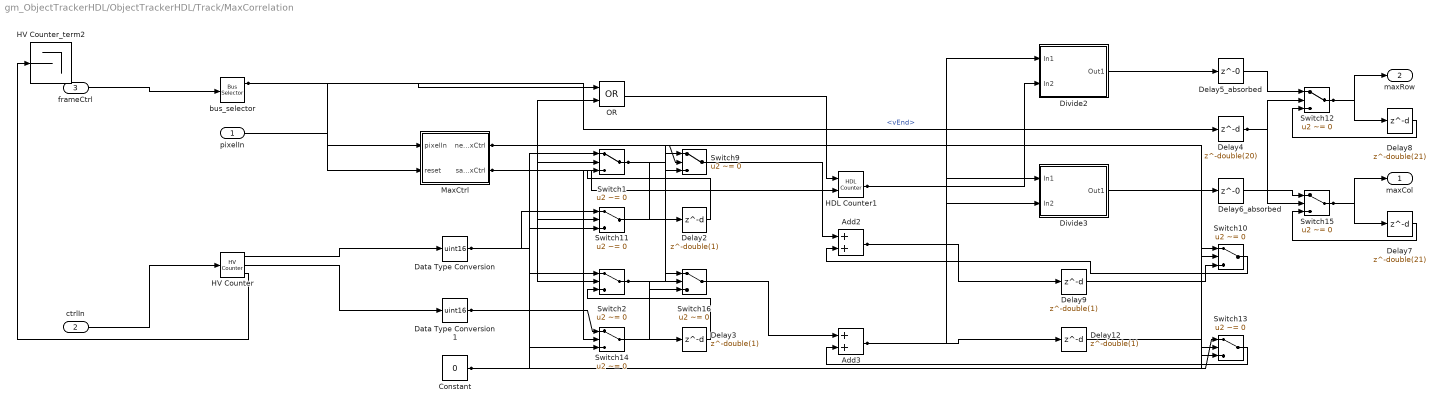
== system gm_ObjectTrackerHDL/ObjectTrackerHDL/Track/MaxCorrelation ==
  pixelIn : Inport  OutDataTypeStr=fixdt(1, 24, 16)  PortDimensions=1  SampleTime=7.94444444444444e-08
  ctrlIn : Inport  Port=2
  frameCtrl : Inport  Port=3
  Add2 : Sum  OutDataTypeStr=uint8  AccumDataTypeStr=uint8  SampleTime=7.94444444444444e-08
  Add3 : Sum  OutDataTypeStr=uint8  AccumDataTypeStr=uint8  SampleTime=7.94444444444444e-08
  Constant : Constant  Value=0  OutDataTypeStr=uint8  SampleTime=7.94444444444444e-08
  Data Type Conversion : DataTypeConversion  OutDataTypeStr=uint16  SampleTime=7.94444444444444e-08  SaturateOnIntegerOverflow=off  RndMeth=Floor
  Data Type Conversion1 : DataTypeConversion  OutDataTypeStr=uint16  SampleTime=7.94444444444444e-08  SaturateOnIntegerOverflow=off  RndMeth=Floor
  Delay{2..3,9,12} (4 alike) : Delay  DelayLength=double(1)  InitialCondition=0  SampleTime=7.94444444444444e-08
  Delay4 : Delay  DelayLength=double(20)  InitialCondition=0  SampleTime=7.94444444444444e-08
  Delay5_absorbed : Delay  DelayLength=0
  Delay6_absorbed : Delay  DelayLength=0
  Delay7 : Delay  DelayLength=double(21)  InitialCondition=0  SampleTime=7.94444444444444e-08
  Delay8 : Delay  DelayLength=double(21)  InitialCondition=0  SampleTime=7.94444444444444e-08
  Divide2 : Subsystem
  Divide3 : Subsystem
  HDL Counter1 : hdlsllib/Sources/HDL Counter  CountType=Free running  CountInit=1  CountStep=1  CountMax=25  CountFromType=Initial value  CountFrom=1  CountResetPort=on  CountLoadPort=off  CountEnbPort=on  CountDirPort=off  CountHitOutputPort=off  CountDataType=Unsigned  CountWordLen=16  CountFracLen=0  CountSampTime=1
  HV Counter : visionhdlutilities/HV Counter  ActivePixelsPerLine=tSize  ActiveVideoLines=tSize  SimulateUsing=Code generation
  HV Counter_term2 : Terminator
  MaxCtrl : Subsystem
  OR : Logic  Operator=OR  AllPortsSameDT=off  OutDataTypeStr=boolean  SampleTime=7.94444444444444e-08
  Switch{1..2,11..12,14..15} (6 alike) : Switch  Criteria=u2 ~= 0  Threshold=double(0)  OutDataTypeStr=uint16  SampleTime=7.94444444444444e-08  SaturateOnIntegerOverflow=off  InputSameDT=off
  Switch{9..10,13,16} (4 alike) : Switch  Criteria=u2 ~= 0  Threshold=double(0)  OutDataTypeStr=uint8  SampleTime=7.94444444444444e-08  SaturateOnIntegerOverflow=off  InputSameDT=off
  bus_selector : BusSelector  OutputSignals=vEnd,vStart
  maxCol : Outport  SampleTime=7.94444444444444e-08
  maxRow : Outport  Port=2  SampleTime=7.94444444444444e-08
  wires:
  pixelIn/1 -> MaxCtrl/1(pixelIn)
  ctrlIn/1 -> HV Counter/1
  frameCtrl/1 -> bus_selector/1
  Add2/1 -> Delay9/1, Divide2/1(In1)
  Add3/1 -> Delay12/1, Divide3/1(In1)
  Constant/1 -> Switch14/3, Switch11/3, Switch13/1, Switch10/1
  Data Type Conversion/1 -> Switch11/1, Switch1/1
  Data Type Conversion1/1 -> Switch14/1, Switch2/1
  Delay4/1 -> Switch15/2, Switch12/2
  HDL Counter1/1 -> Divide2/2(In2), Divide3/2(In2)
  HV Counter/1 -> Data Type Conversion/1
  HV Counter/2 -> Data Type Conversion1/1
  HV Counter/3 -> HV Counter_term2/1
  MaxCtrl/1(newMaxCtrl) -> Switch9/2, Switch16/2, OR/2, Switch2/2, Switch13/2, Switch1/2, Switch10/2
  MaxCtrl/2(sameMaxCtrl) -> Switch14/2, Switch11/2, HDL Counter1/2
  OR/1 -> HDL Counter1/1
  bus_selector/1 -> OR/1, Delay4/1, MaxCtrl/2(reset)  "<vEnd>"
  Switch1/1 -> Switch9/1, Delay2/1
  Switch11/1 -> Switch9/3
  Switch12/1 -> maxRow/1, Delay8/1
  Switch14/1 -> Switch16/3
  Switch15/1 -> maxCol/1, Delay7/1
  Switch2/1 -> Switch16/1, Delay3/1
  Delay8/1 -> Switch12/3
  Delay5_absorbed/1 -> Switch12/1
  Delay3/1 -> Switch2/3
  Delay12/1 -> Switch13/3
  Switch16/1 -> Add3/1
  Switch13/1 -> Add3/2
  Delay7/1 -> Switch15/3
  Delay6_absorbed/1 -> Switch15/1
  Delay2/1 -> Switch1/3
  Delay9/1 -> Switch10/3
  Switch9/1 -> Add2/1
  Switch10/1 -> Add2/2
  Divide3/1(Out1) -> Delay6_absorbed/1
  Divide2/1(Out1) -> Delay5_absorbed/1
